simulink model "main"  (R2024a)
settings: Solver=VariableStepAuto  StartTime=0.0  StopTime=100  RelTol=1e-3
settings Model: Creator=filip  LastModifiedBy=filip

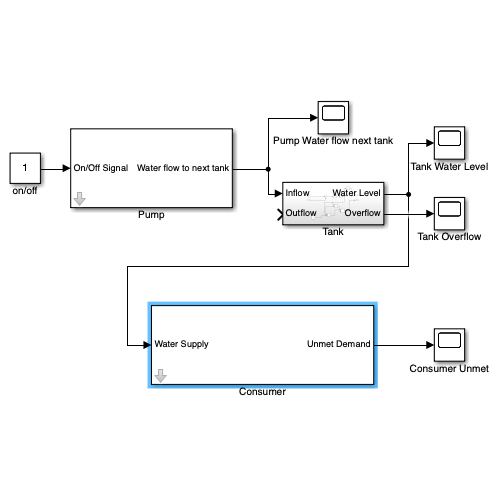
[thumbnail: Simulink's stored preview of the top-level diagram]
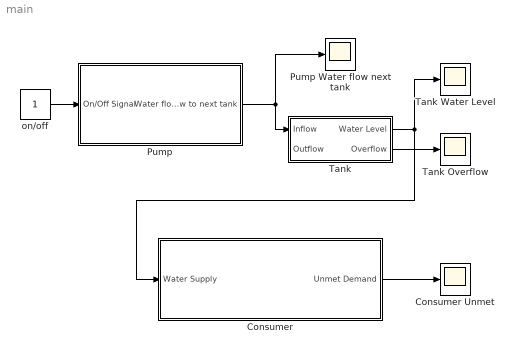
== system main ==
  Consumer : Subsystem  mask{a_i=5, f_i=1, d_i=20}
  Consumer Unmet : Scope
  Pump : Subsystem  mask{p_i=200}
  Pump Water flow next tank : Scope
  Tank : Subsystem
  Tank Overflow : Scope
  Tank Water Level : Scope
  on/off : Constant
  wires:
  Pump/1(Water flow to next tank) -> Tank/1(Inflow), Pump Water flow next tank/1
  on/off/1 -> Pump/1(On/Off Signal)
  Tank/1(Water Level) -> Tank Water Level/1, Consumer/1(Water Supply)
  Tank/2(Overflow) -> Tank Overflow/1
  Consumer/1(Unmet Demand) -> Consumer Unmet/1

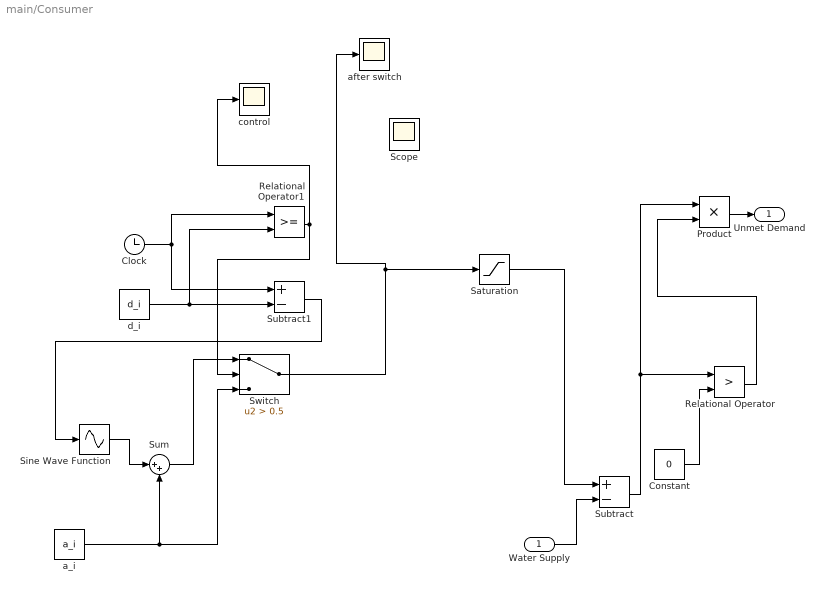
== system main/Consumer ==
  Water Supply : Inport
  Clock : Clock
  Constant : Constant  Value=0
  Product : Product
  Relational Operator : RelationalOperator  Operator=>  OutDataTypeStr=boolean  RndMeth=Simplest  InputSameDT=off
  Relational Operator1 : RelationalOperator  OutDataTypeStr=boolean  RndMeth=Simplest  InputSameDT=off
  Saturation : Saturate  UpperLimit=inf  LowerLimit=0
  Scope : Scope
  Sine Wave Function : Sin  TimeSource=Use external signal  Amplitude=a_i  Frequency=f_i  SampleTime=0
  Subtract : Sum  Inputs=+-
  Subtract1 : Sum  Inputs=+-
  Sum : Sum  Inputs=|++
  Switch : Switch  Criteria=u2 > Threshold  Threshold=0.5  SaturateOnIntegerOverflow=off  InputSameDT=off
  a_i : Constant  Value=a_i
  after switch : Scope
  control : Scope
  d_i : Constant  Value=d_i
  Unmet Demand : Outport
  wires:
  a_i/1 -> Sum/2, Switch/3
  Water Supply/1 -> Subtract/2
  Subtract/1 -> Relational Operator/1, Product/1
  Relational Operator/1 -> Product/2
  Product/1 -> Unmet Demand/1
  Switch/1 -> after switch/1, Saturation/1
  Saturation/1 -> Subtract/1
  Constant/1 -> Relational Operator/2
  Clock/1 -> Relational Operator1/1, Subtract1/1
  d_i/1 -> Relational Operator1/2, Subtract1/2
  Subtract1/1 -> Sine Wave Function/1
  Relational Operator1/1 -> Switch/2, control/1
  Sum/1 -> Switch/1
  Sine Wave Function/1 -> Sum/1

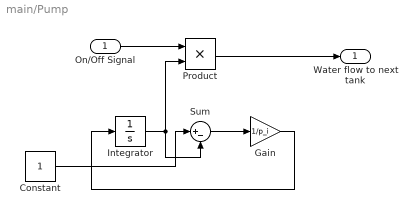
== system main/Pump ==
  On/Off Signal : Inport
  Constant : Constant
  Gain : Gain  Gain=1/p_i
  Integrator : Integrator
  Product : Product
  Sum : Sum  Inputs=|+-
  Water flow to next tank : Outport
  wires:
  Integrator/1 -> Product/2, Sum/2
  On/Off Signal/1 -> Product/1
  Product/1 -> Water flow to next tank/1
  Constant/1 -> Sum/1
  Sum/1 -> Gain/1
  Gain/1 -> Integrator/1

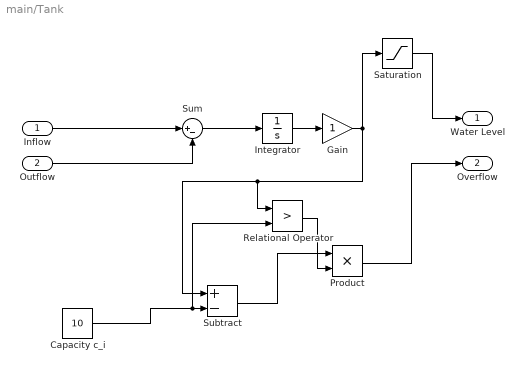
== system main/Tank ==
  Inflow : Inport
  Outflow : Inport  Port=2
  Capacity c_i : Constant  Value=10
  Gain : Gain
  Integrator : Integrator
  Product : Product
  Relational Operator : RelationalOperator  Operator=>  OutDataTypeStr=boolean  RndMeth=Simplest  InputSameDT=off
  Saturation : Saturate  UpperLimit=10  LowerLimit=0
  Subtract : Sum  Inputs=+-
  Sum : Sum  Inputs=|+-
  Water Level : Outport
  Overflow : Outport  Port=2
  wires:
  Inflow/1 -> Sum/1
  Outflow/1 -> Sum/2
  Sum/1 -> Integrator/1
  Integrator/1 -> Gain/1
  Gain/1 -> Relational Operator/1, Subtract/1, Saturation/1
  Capacity c_i/1 -> Relational Operator/2, Subtract/2
  Saturation/1 -> Water Level/1
  Product/1 -> Overflow/1
  Subtract/1 -> Product/1
  Relational Operator/1 -> Product/2
